simulink model "GEN__S3_1_PI"  (R2024a)
settings: Solver=VariableStepAuto  StartTime=0.0  StopTime=10.0  RelTol=1e-3
settings Model: Creator=edub  LastModifiedBy=edub

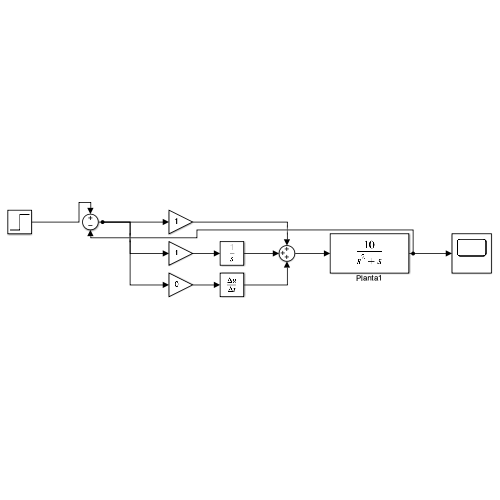
[thumbnail: Simulink's stored preview of the top-level diagram]
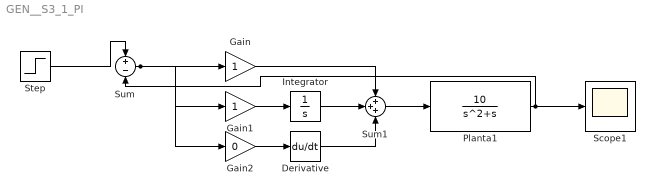
== system GEN__S3_1_PI ==
  Derivative : Derivative
  Gain : Gain
  Gain1 : Gain
  Gain2 : Gain  Gain=0
  Integrator : Integrator
  Planta1 : TransferFcn  Numerator=[0 0 10]  Denominator=[1 1 0]
  Scope1 : Scope
  Step : Step  SampleTime=0
  Sum : Sum  Inputs=+-
  Sum1 : Sum  Inputs=+++
  wires:
  Step/1 -> Sum/1
  Sum/1 -> Gain/1, Gain1/1, Gain2/1
  Gain/1 -> Sum1/1
  Gain1/1 -> Integrator/1
  Integrator/1 -> Sum1/2
  Gain2/1 -> Derivative/1
  Derivative/1 -> Sum1/3
  Sum1/1 -> Planta1/1
  Planta1/1 -> Scope1/1, Sum/2
